simulink model "horizontal_sim"  (R2019b)
settings: Solver=VariableStepAuto  StartTime=0.0  StopTime=10.0  RelTol=1e-3
values from neighbouring files (symbols this model uses):
  Fs = Fl-Fr    [main_rocketmodel.m]    (also in main_sim_rocket.m; rocket_model.m)
  m = 549054    [main_rocketmodel.m]    (also in main_sim_rocket.m; rocket_model.m = 25.4; sim_lin.m; test_bangbang.m)
  phi = (1e-6)*square(t_signal,25)    [main_rocketmodel.m]    (also in main_sim_rocket.m = zeros(length(t_signal),1); nominal_trajectory.m = zeros(length(t_signal),1); rocket_model.m = out.phi; sim_lin.m)
  theta = 0    [main_rocketmodel.m]    (also in main_sim_rocket.m; rocket_model.m)
settings Model: Creator=bia  LastModifiedBy=bia

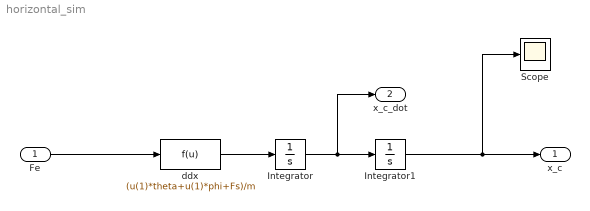
== system horizontal_sim ==
  Fe : Inport
  Integrator : Integrator  ContinuousStateAttributes='x_c_dot'
  Integrator1 : Integrator  ContinuousStateAttributes='x_c'
  Scope : Scope
  ddx : Fcn  Expr=(u(1)*theta+u(1)*phi+Fs)/m
  x_c : Outport
  x_c_dot : Outport  Port=2
  wires:
  Integrator/1 -> x_c_dot/1, Integrator1/1
  Fe/1 -> ddx/1
  Integrator1/1 -> Scope/1, x_c/1
  ddx/1 -> Integrator/1
